simulink model "MTT1"  (Simulink 8.5)
settings: Solver=ode45  StartTime=0.0  StopTime=100  RelTol=1e-3
values from neighbouring files (symbols this model uses):
  map = createWorld(city_width, building_height, num_blocks, street_width)    [param.m]
undefined symbols (not defined in the file or in its folder): camera_multi_target, drawMultipleAircraftTargets, drawTargetsAndCov, geolocationMultiTargetGimCont2, P, point_gimbal, SelectedTarget1, target_follow, TargetSelectionSingleUAV
settings Model: Creator=Rajnikant.Sharma  LastModifiedBy=fkv344
settings DebuggingCC: SolverPrmCheckMsg=warning  FcnCallInpInsideContextMsg=EnableAllAsWarning

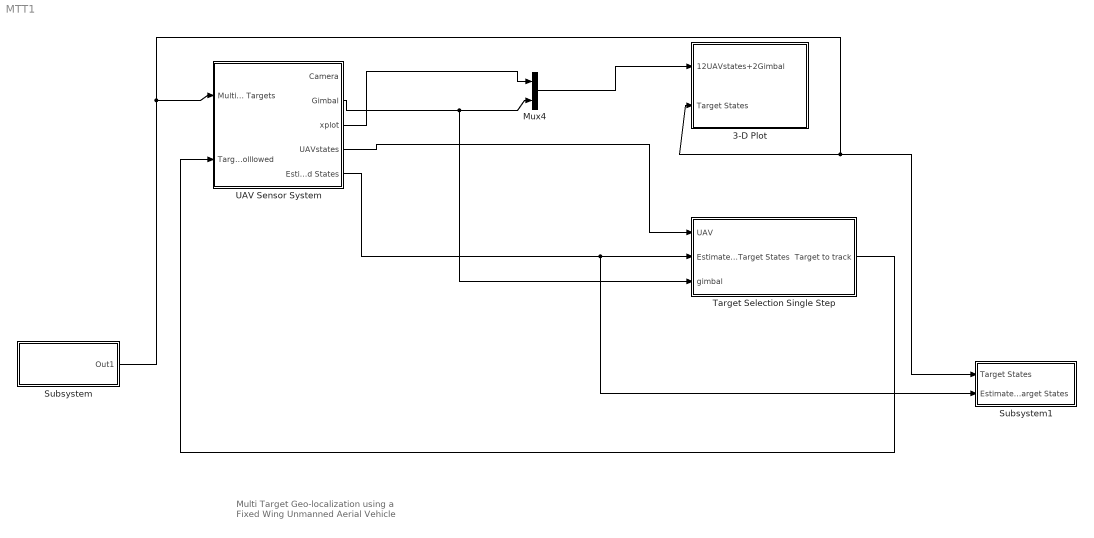
== system MTT1 ==
  note: Multi Target Geo-localization using a
      | Fixed Wing Unmanned Aerial Vehicle
  3-D Plot : Subsystem  mask{cam_fov=P.cam_fov, R_min=P.R_min, map=map, NOT=3, NOU=1}
      mask prompts: cam_fov "FOV of Camera"; NOT "Number of Targets"; NOU "Number of UAVs"
      mask init:
      | % parameters for drawing aircraft
      |   % scale size
      |   size = 2;
      |   fuse_l1    = 7;
      |   fuse_l2    = 4;
      |   fuse_l3    = 15;
      |   fuse_w     = 2;
      |   wing_l     = 6;
      |   wing_w     = 20;
      |   tail_l     = 3;
      |   tail_h     = 3;
      |   tailwing_w = 10;
      |   tailwing_l = 3;
      |   % colors
      |   red     = [1, 0, 0];
      |   green   = [0, 1, 0];
      |   blue    = [0, 0, 1];
      |   yellow  = [1,1,0];
      |   magenta = [0, 1, 1];
      |   
      | 
      | % define vertices and faces for aircraft
      |   V = [...
      |     fuse_l1,             0,             0;...        % point 1
      |     fuse_l2,            -fuse_w/2,     -fuse_w/2;... % point 2     
      |     fuse_l2,             fuse_w/2,     -fuse_w/2;... % point 3     
      |     fuse_l2,             fuse_w/2,      fuse_w/2;... % point 4
      |     fuse_l2,            -fuse_w/2,      fuse_w/2;... % point 5
      |    -fuse_l3,             0,             0;...        % point 6
      |     0,                   wing_w/2,      0;...        % point 7
      |    -wing_l,              wing_w/2,      0;...        % point 8
      |    -wing_l,             -wing_w/2,      0;...        % point 9
      |     0,                  -wing_w/2,      0;...        % point 10
      |    -fuse_l3+tailwing_l,  tailwing_w/2,  0;...        % point 11
      |    -fuse_l3,             tailwing_w/2,  0;...        % point 12
      |    -fuse_l3,            -tailwing_w/2,  0;...        % point 13
      |    -fuse_l3+tailwing_l, -tailwing_w/2,  0;...        % point 14
      |    -fuse_l3+tailwing_l,  0,             0;...        % point 15
      |    -fuse_l3+tailwing_l,  0,             -tail_h;...  % point 16
      |    -fuse_l3,             0,             -tail_h;...  % point 17
      |   ];
      |   
      |   F = [...
      |         1,  2,  3,  1;... % nose-top
      |         1,  3,  4,  1;... % nose-left
      |         1,  4,  5,  1;... % nose-bottom
      |         1,  5,  2,  1;... % nose-right
      |         2,  3,  6,  2;... % fuselage-top
      |         3,  6,  4,  3;... % fuselage-left
      |         4,  6,  5,  4;... % fuselage-bottom
      |         2,  5,  6,  2;... % fuselage-right
      |         7,  8,  9, 10;... % wing
      |        11, 12, 13, 14;... % tailwing
      |         6, 15, 17, 17;... % tail
      |         
      |   ];  
      |   
      |   colors = [...
      |         yellow;... % nose-top
      |         yellow;... % nose-left
      |         yellow;... % nose-bottom
      |         yellow;... % nose-right
      |         blue;... % fuselage-top
      |         blue;... % fuselage-left
      |         red;... % fuselage-bottom
      |         blue;... % fuselage-right
      |         green;... % wing
      |         green;... % tailwing
      |         blue;... % tail
      |     ];
      | 
      |   V = size*V;   % rescale vertices
      |   Vt=[];
      |   Ft=[];
  Mux4 : Mux  Inputs=2
  Subsystem : Subsystem
  Subsystem1 : Subsystem  mask{map=map, NOT=3}
      mask prompts: NOT "Number of Targets"
      mask init: same as MTT1/3-D Plot
  Target Selection Single Step : Subsystem  mask{P=P, nt=3, k=1, nu=1}
      mask prompts: P "Parameters"; nt "number of targets"; k "number of steps"; nu "number of uavs"
  UAV Sensor System : Subsystem  mask{nt=3, P=P}
      mask prompts: nt "number of targets"; P "parameters"
  wires:
  Subsystem/1(Out1) -> UAV Sensor System/1(Multiple Targets), 3-D Plot/2(Target States), Subsystem1/1(Target States)
  Target Selection Single Step/1(Target to track) -> UAV Sensor System/2(Target to folllowed)
  UAV Sensor System/5(Estimated States) -> Target Selection Single Step/2(Estimated Target States), Subsystem1/2(Estimated Target States)
  UAV Sensor System/3(xplot) -> Mux4/1
  UAV Sensor System/2(Gimbal) -> Mux4/2, Target Selection Single Step/3(gimbal)
  UAV Sensor System/4(UAVstates) -> Target Selection Single Step/1(UAV)
  Mux4/1 -> 3-D Plot/1(12UAVstates+2Gimbal)

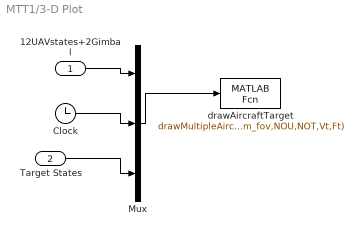
== system MTT1/3-D Plot ==
  12UAVstates+2Gimbal : Inport
  Target States : Inport  Port=2
  Clock : Clock
  Mux : Mux  Inputs=3
  drawAircraftTarget : MATLABFcn  MATLABFcn=drawMultipleAircraftTargets(u,V,F,colors,map,R_min,cam_fov,NOU,NOT,Vt,Ft)  OutputDimensions=0  SampleTime=P.Ts
  wires:
  Clock/1 -> Mux/2
  12UAVstates+2Gimbal/1 -> Mux/1
  Mux/1 -> drawAircraftTarget/1
  Target States/1 -> Mux/3

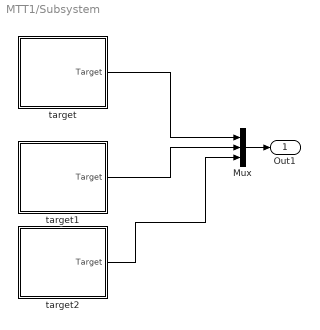
== system MTT1/Subsystem ==
  Mux : Mux  Inputs=3
  target : Subsystem  mask{P=P, z0=[0;200;0], v0=[P.target_velocity; 0; 0];, map=map}
      mask prompts: P "parameters"; z0 "iitial position"; v0 "initial velocity"
      mask Display: image(imread('monstertruck.jpg'))
  target1 : Subsystem  mask{P=P, z0=[100;200;0], v0=[P.target_velocity; 0; 0];, map=map}
      mask prompts: P "parameters"; z0 "iitial position"; v0 "initial velocity"
      mask Display: image(imread('monstertruck.jpg'))
  target2 : Subsystem  mask{P=P, z0=[100;100;0], v0=[P.target_velocity; 0; 0];, map=map}
      mask prompts: P "parameters"; z0 "iitial position"; v0 "initial velocity"
      mask Display: image(imread('monstertruck.jpg'))
  Out1 : Outport
  wires:
  target/1(Target) -> Mux/1
  target1/1(Target) -> Mux/2
  target2/1(Target) -> Mux/3
  Mux/1 -> Out1/1

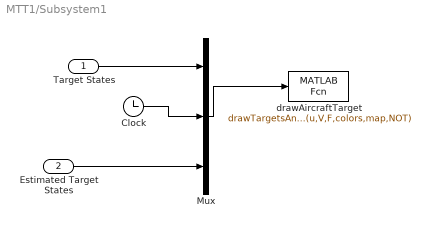
== system MTT1/Subsystem1 ==
  Target States : Inport
  Estimated Target States : Inport  Port=2
  Clock : Clock
  Mux : Mux  Inputs=3
  drawAircraftTarget : MATLABFcn  MATLABFcn=drawTargetsAndCov(u,V,F,colors,map,NOT)  OutputDimensions=0  SampleTime=0.1
  wires:
  Mux/1 -> drawAircraftTarget/1
  Target States/1 -> Mux/1
  Estimated Target States/1 -> Mux/3
  Clock/1 -> Mux/2

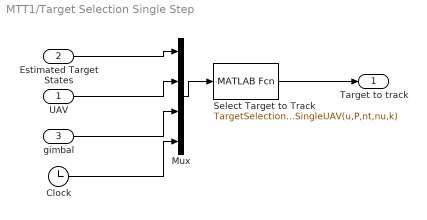
== system MTT1/Target Selection Single Step ==
  UAV : Inport
  Estimated Target States : Inport  Port=2
  gimbal : Inport  Port=3
  Clock : Clock
  Mux : Mux
  Select Target to Track : MATLABFcn  MATLABFcn=TargetSelectionSingleUAV(u,P,nt,nu,k)  OutputDimensions=1  SampleTime=P.Tg
  Target to track : Outport
  wires:
  Select Target to Track/1 -> Target to track/1
  Mux/1 -> Select Target to Track/1
  gimbal/1 -> Mux/3
  Estimated Target States/1 -> Mux/1
  UAV/1 -> Mux/2
  Clock/1 -> Mux/4

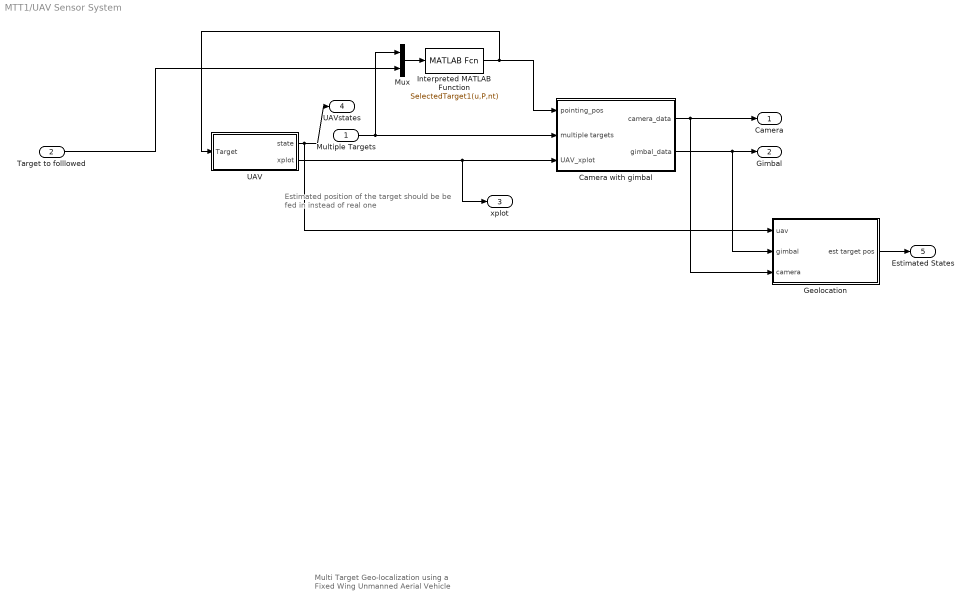
== system MTT1/UAV Sensor System ==
  note: Estimated position of the target should be
      | be fed in instead of real one
  note: Multi Target Geo-localization using a
      | Fixed Wing Unmanned Aerial Vehicle
  Multiple Targets : Inport
  Target to folllowed : Inport  Port=2
  Camera with gimbal : Subsystem
  Geolocation : Subsystem  mask{P=P, nt=3}
      mask prompts: P "Parameters"; nt "Number of Targets"
  Interpreted MATLAB Function : MATLABFcn  MATLABFcn=SelectedTarget1(u,P,nt)  OutputDimensions=6  SampleTime=P.Tg
  Mux : Mux  Inputs=2
  UAV : Subsystem
  "Camera " : Outport
  Gimbal : Outport  Port=2
  xplot : Outport  Port=3
  UAVstates : Outport  Port=4
  Estimated States : Outport  Port=5
  wires:
  UAV/2(xplot) -> Camera with gimbal/3(UAV_xplot), xplot/1
  Multiple Targets/1 -> Camera with gimbal/2(multiple targets), Mux/1
  Camera with gimbal/1(camera_data) -> "Camera "/1, Geolocation/3(camera)
  Camera with gimbal/2(gimbal_data) -> Gimbal/1, Geolocation/2(gimbal)
  UAV/1(state) -> UAVstates/1, Geolocation/1(uav)
  Mux/1 -> Interpreted MATLAB Function/1
  Target to folllowed/1 -> Mux/2
  Interpreted MATLAB Function/1 -> Camera with gimbal/1(pointing_pos), UAV/1(Target)
  Geolocation/1(est target pos) -> Estimated States/1

== system MTT1/Subsystem/target ==
  S-Function : S-Function  FunctionName=target_motion_Init  Parameters=P,map,z0,v0
  Target : Outport
  wires:
  S-Function/1 -> Target/1

== system MTT1/Subsystem/target1 ==
  S-Function : S-Function  FunctionName=target_motion_Init  Parameters=P,map,z0,v0
  Target : Outport
  wires:
  S-Function/1 -> Target/1

== system MTT1/Subsystem/target2 ==
  S-Function : S-Function  FunctionName=target_motion_Init  Parameters=P,map,z0,v0
  Target : Outport
  wires:
  S-Function/1 -> Target/1

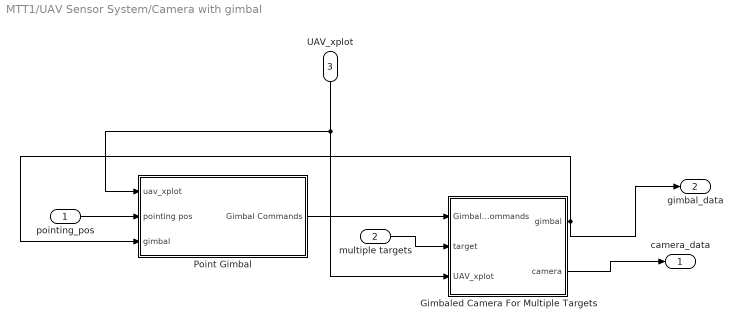
== system MTT1/UAV Sensor System/Camera with gimbal ==
  pointing_pos : Inport
  multiple targets : Inport  Port=2
  UAV_xplot : Inport  Port=3
  Gimbaled Camera For Multiple Targets : Subsystem  mask{P=P, NOT=3}
      mask prompts: P "Parameters"; NOT "Number of Targets"
  Point Gimbal : Subsystem
  camera_data : Outport
  gimbal_data : Outport  Port=2
  wires:
  Gimbaled Camera For Multiple Targets/1(gimbal) -> Point Gimbal/3(gimbal), gimbal_data/1
  Point Gimbal/1(Gimbal Commands) -> Gimbaled Camera For Multiple Targets/1(Gimbal Commands)
  Gimbaled Camera For Multiple Targets/2(camera) -> camera_data/1
  multiple targets/1 -> Gimbaled Camera For Multiple Targets/2(target)
  pointing_pos/1 -> Point Gimbal/2(pointing pos)
  UAV_xplot/1 -> Point Gimbal/1(uav_xplot), Gimbaled Camera For Multiple Targets/3(UAV_xplot)

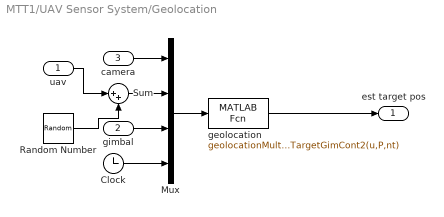
== system MTT1/UAV Sensor System/Geolocation ==
  uav : Inport
  gimbal : Inport  Port=2
  camera : Inport  Port=3
  Clock : Clock
  Mux : Mux
  Random Number : RandomNumber  Mean=zeros(16,1)  Variance=[P.sigma_measurement_n; P.sigma_measurement_e; P.sigma_measurement_h;zeros(3,1);0.0*ones(3,1);zeros(7,1)]  SampleTime=0.1
  Sum : Sum  Inputs=|++
  geolocation : MATLABFcn  MATLABFcn=geolocationMultiTargetGimCont2(u,P,nt)  OutputDimensions=30*nt  SampleTime=P.Tc
  est target pos : Outport
  wires:
  Clock/1 -> Mux/4
  gimbal/1 -> Mux/3
  camera/1 -> Mux/1
  geolocation/1 -> est target pos/1
  Mux/1 -> geolocation/1
  uav/1 -> Sum/1
  Random Number/1 -> Sum/2
  Sum/1 -> Mux/2

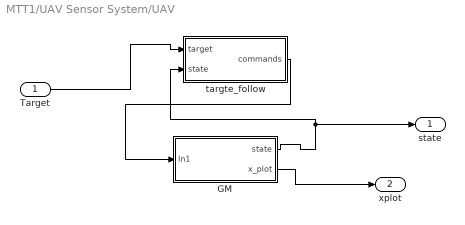
== system MTT1/UAV Sensor System/UAV ==
  Target : Inport
  GM : Subsystem  mask{pn0=20, pe0=200, pd0=-100, Va0=P.Va0, psi0=P.psi0, P=P}
      mask prompts: pn0 "nortth"; pe0 "east"; pd0 "altitude"; Va0 "airspeed"; psi0 "COurse Angle"; P "UAV Parameters"
  targte_follow : Subsystem  mask{P=P, h_d=100, Va_d=P.Va0, flag=2}
      mask prompts: P "Parameters"; h_d "height"; Va_d "airspeed"
  state : Outport
  xplot : Outport  Port=2
  wires:
  GM/1(state) -> targte_follow/2(state), state/1
  targte_follow/1(commands) -> GM/1(In1)
  Target/1 -> targte_follow/1(target)
  GM/2(x_plot) -> xplot/1

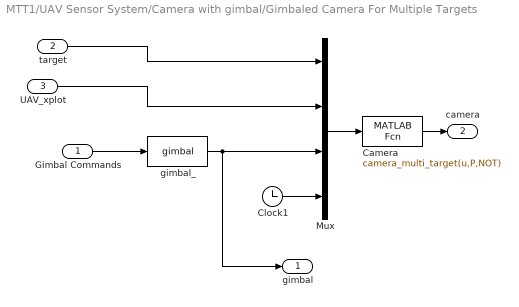
== system MTT1/UAV Sensor System/Camera with gimbal/Gimbaled Camera For Multiple Targets ==
  Gimbal Commands : Inport
  target : Inport  Port=2
  UAV_xplot : Inport  Port=3
  Camera : MATLABFcn  MATLABFcn=camera_multi_target(u,P,NOT)  OutputDimensions=3*NOT  SampleTime=1/P.cam_fps
  Clock1 : Clock
  Mux : Mux
  gimbal_ : S-Function  FunctionName=gimbal  Parameters=P
  gimbal : Outport
  camera : Outport  Port=2
  wires:
  Mux/1 -> Camera/1
  UAV_xplot/1 -> Mux/2
  Camera/1 -> camera/1
  target/1 -> Mux/1
  Clock1/1 -> Mux/4
  Gimbal Commands/1 -> gimbal_/1
  gimbal_/1 -> Mux/3, gimbal/1

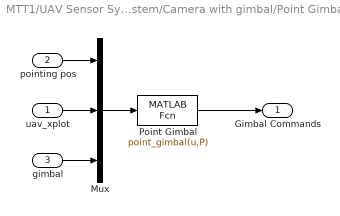
== system MTT1/UAV Sensor System/Camera with gimbal/Point Gimbal ==
  uav_xplot : Inport
  pointing pos : Inport  Port=2
  gimbal : Inport  Port=3
  Mux : Mux  Inputs=3
  Point Gimbal : MATLABFcn  MATLABFcn=point_gimbal(u,P)  OutputDimensions=2  SampleTime=P.Ts
  Gimbal Commands : Outport
  wires:
  Mux/1 -> Point Gimbal/1
  uav_xplot/1 -> Mux/2
  Point Gimbal/1 -> Gimbal Commands/1
  pointing pos/1 -> Mux/1
  gimbal/1 -> Mux/3

== system MTT1/UAV Sensor System/UAV/GM ==
  In1 : Inport
  Demux : Demux  Outputs=[16;12]
  S-Function : S-Function  FunctionName=guidance_model_new  Parameters=P,pn0,pe0,pd0,psi0,Va0
  state : Outport
  x_plot : Outport  Port=2
  wires:
  Demux/1 -> state/1
  Demux/2 -> x_plot/1
  S-Function/1 -> Demux/1
  In1/1 -> S-Function/1

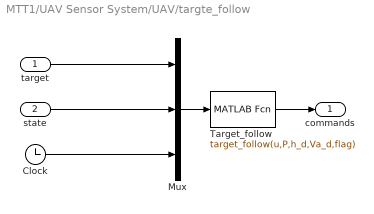
== system MTT1/UAV Sensor System/UAV/targte_follow ==
  target : Inport
  state : Inport  Port=2
  Clock : Clock
  Mux : Mux  Inputs=3
  Target_follow : MATLABFcn  MATLABFcn=target_follow(u,P,h_d,Va_d,flag)  OutputDimensions=3  SampleTime=P.Ts
  commands : Outport
  wires:
  state/1 -> Mux/2
  Clock/1 -> Mux/3
  target/1 -> Mux/1
  Mux/1 -> Target_follow/1
  Target_follow/1 -> commands/1
